simulink model "MotorSpeedModeling"  (R2015b)
settings: Solver=VariableStepAuto  StartTime=0.0  StopTime=10.0  RelTol=1e-3
values from neighbouring files (symbols this model uses):
  b = str2num(get(handles.frictionText,'String'))    [MotorSpeedSimulinkModeling.m]
  J = str2num(get(handles.inertiaText,'String'))    [MotorSpeedSimulinkModeling.m]
  Ke = str2num(get(handles.emfText,'String'))    [MotorSpeedSimulinkModeling.m]
  Kt = str2num(get(handles.torqueText,'String'))    [MotorSpeedSimulinkModeling.m]
  L = str2num(get(handles.inductionText,'String'))    [MotorSpeedSimulinkModeling.m]
  R = str2num(get(handles.resistanceText,'String'))    [MotorSpeedSimulinkModeling.m]
settings Model: Creator=YOUNG  LastModifiedBy=YOUNG

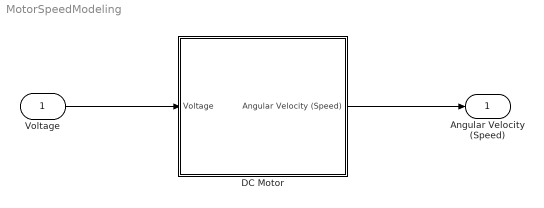
== system MotorSpeedModeling ==
  Voltage : Inport
  DC Motor : Subsystem
      mask Display: image(imread('dc_motor_diagram.png'));
  Angular Velocity (Speed) : Outport
  wires:
  Voltage/1 -> DC Motor/1(Voltage)
  DC Motor/1(Angular Velocity (Speed)) -> Angular Velocity (Speed)/1

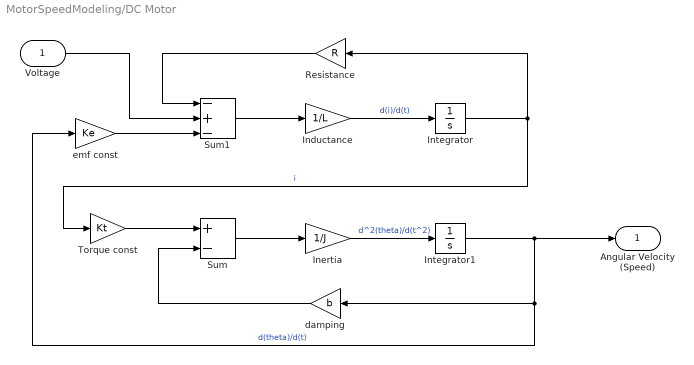
== system MotorSpeedModeling/DC Motor ==
  Voltage : Inport
  Inductance : Gain  Gain=1/L
  Inertia : Gain  Gain=1/J
  Integrator : Integrator
  Integrator1 : Integrator
  Resistance : Gain  Gain=R
  Sum : Sum  Inputs=+-
  Sum1 : Sum  Inputs=-+-
  Torque const : Gain  Gain=Kt
  damping : Gain  Gain=b
  emf const : Gain  Gain=Ke
  Angular Velocity (Speed) : Outport
  wires:
  damping/1 -> Sum/2
  Resistance/1 -> Sum1/1
  Inductance/1 -> Integrator/1  "d(i)/d(t)"
  Integrator/1 -> Torque const/1, Resistance/1  "i"
  emf const/1 -> Sum1/3
  Voltage/1 -> Sum1/2
  Sum/1 -> Inertia/1
  Torque const/1 -> Sum/1
  Sum1/1 -> Inductance/1
  Inertia/1 -> Integrator1/1  "d^2(theta)/d(t^2)"
  Integrator1/1 -> Angular Velocity (Speed)/1, damping/1, emf const/1  "d(theta)/d(t)"
